simulink model "PRBS_Gen"  (R2019a)
settings: Solver=FixedStepAuto  StartTime=0.0  StopTime=TSim  FixedStep=0.2  RelTol=1e-3
values from neighbouring files (symbols this model uses):
  Num_Switch = 50    [MissionBlocks.m]    (also in Test.m = 1)
  Percent = 0.1    [MissionBlocks.m]    (also in Test.m)
  Samp_end = 2    [MissionBlocks.m]    (also in Test.m)
  Samp_start = 100    [MissionBlocks.m]    (also in Test.m)
  Samp_Switch = 2    [MissionBlocks.m]    (also in Test.m = 1000)
  Wf = [0.01335 0.01669 0.02 0.025 0.03 0.0334 0.04172 0.05 0.05841 0.06676]    [MissionBlocks.m]    (also in Test.m = WfMtx(2))
libraries: Lib_Solve_ModelSource_TMATS x1
settings Model: Creator=anton  LastModifiedBy=anton

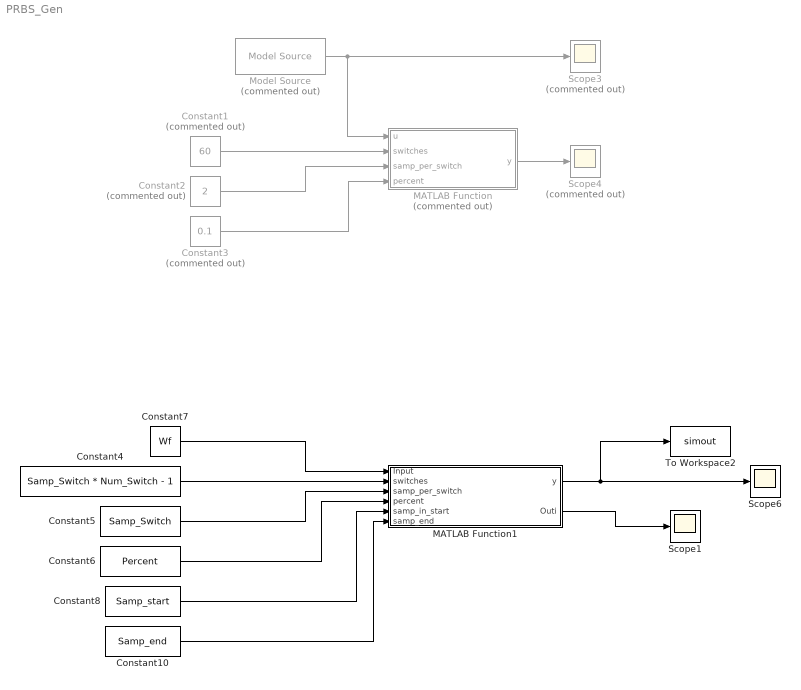
== system PRBS_Gen ==
  Constant1 : Constant  Commented=on  Value=60
  Constant10 : Constant  Value=Samp_end
  Constant2 : Constant  Commented=on  Value=2
  Constant3 : Constant  Commented=on  Value=0.1
  Constant4 : Constant  Value=Samp_Switch * Num_Switch - 1
  Constant5 : Constant  Value=Samp_Switch
  Constant6 : Constant  Value=Percent
  Constant7 : Constant  Value=Wf
  Constant8 : Constant  Value=Samp_start
  MATLAB Function : MATLAB Function  Commented=on  TreatAsAtomicUnit=on
  MATLAB Function1 : MATLAB Function  TreatAsAtomicUnit=on
  Model Source : Lib_Solve_ModelSource_TMATS/Model Source  Commented=on  T_vec_M=[0 15 15.1 30 30.1 45]  input_array_M=[5 5 10 10 15 15 ]
  Scope1 : Scope
  Scope3 : Scope  Commented=on
  Scope4 : Scope  Commented=on
  Scope6 : Scope
  To Workspace2 : ToWorkspace  VariableName=simout  SaveFormat=Timeseries  SampleTime=-1
  wires:
  Model Source/1 -> MATLAB Function/1(u), Scope3/1
  MATLAB Function/1(y) -> Scope4/1
  Constant1/1 -> MATLAB Function/2(switches)
  Constant2/1 -> MATLAB Function/3(samp_per_switch)
  Constant3/1 -> MATLAB Function/4(percent)
  Constant6/1 -> MATLAB Function1/4(percent)
  Constant5/1 -> MATLAB Function1/3(samp_per_switch)
  Constant4/1 -> MATLAB Function1/2(switches)
  MATLAB Function1/1(y) -> To Workspace2/1, Scope6/1
  Constant7/1 -> MATLAB Function1/1(Input)
  Constant8/1 -> MATLAB Function1/5(samp_in_start)
  Constant10/1 -> MATLAB Function1/6(samp_end)
  MATLAB Function1/2(Outi) -> Scope1/1

== matlab function PRBS_Gen/MATLAB Function1 ==
  settings: updateMethod=DISCRETE  sampleTime=0.2
  data: Input input; y output; switches input; samp_per_switch input; percent input; samp_in_start input; samp_end input; Outi output
function [y,Outi] = fcn(Input,switches,samp_per_switch,percent,samp_in_start,samp_end)
     
persistent state;
persistent u;
persistent switch_count;
persistent switch_stay;
persistent level_count;
persistent output

persistent i;

%Initiates outputs
y = Input(1);
LengIn = length(Input);
Outi = 0;

%Initiates persistent variables
if isempty(state)

    state = 0;
    switch_count = 0;
    switch_stay = 0;
    level_count = 1;
    output = Input(1);
    u = Input(1);
    i = 0;

    return;

end

switch state
    case 0
        %Updates output
        output = u;
        %Updates the number of samples of signal holding
        switch_stay = switch_stay + 1;
        %Verifies if signal has been held for enought sample periods
        if switch_stay == samp_in_start
            state = 1;
            switch_stay = samp_per_switch;
        end
    case 1
        %Verifies if signal has been held for enought sample periods
        if switch_stay == samp_per_switch && switch_count <= switches
            %Generates a random numver for coefficient generation
            coeff = rand(1,1);
            %Determines the coefficient for oscilation around input value
            if coeff > 0.5
                coeff = 1;
            else
                coeff = -1;
            end
            %Updates output
            output = u * (1 + coeff * percent);
            switch_stay = 0;
            i = i+1;
        end
        
        %Updates switch count
        switch_stay = switch_stay + 1;
        switch_count = switch_count + 1;
        
        %All switches have been accomplisehd
        if switch_count > switches
            state = 2;
            switch_stay = 0;
            switch_count = 0;
            i = 0;
        end
        
    case 2
        %If number of switches have been reached, the output must remain
        %equal current input level
        output = u;
        %Updates switch count
        switch_stay = switch_stay + 1;
        %If output is at current lavel for enough samples, next state is
        %activated
        if switch_stay >= samp_end
            state = 3;
            switch_stay = 0;
        end
        %If change is deteced, cycle starts again
    case 3
        %Updates signal level counter
        level_count = level_count + 1;
        %Updates u for next input level if possible
        if level_count <= LengIn
            u = Input(level_count);
            state = 0;
        end
        
end

%Updates fuel level for mission
y = output;
%Updates i - shows how many times the output is calculated while in prbs
Outi = i;

== matlab function PRBS_Gen/MATLAB Function ==
  settings: updateMethod=DISCRETE  sampleTime=0.2
  data: u input; y output; switches input; samp_per_switch input; percent input
function y = fcn(u,switches,samp_per_switch,percent)

persistent change;     %detects change in input
persistent state;
persistent switch_count;
persistent switch_stay;
persistent uk1
persistent output

y = 0;

if isempty(change)

    change = 1;
    state = 0;
    switch_count = 0;
    switch_stay = 0;
    uk1 = u;
    output = 0;

    return;

end



switch state
    case 0
        %Updates output
        output = u;
        %Updates the number of samples of signal holding
        switch_stay = switch_stay + 1;
        %Verifies if signal has been held for enought sample periods
        if switch_stay == samp_per_switch
            state = 1;
        end
    case 1
        %Verifies if signal has been held for enought sample periods
        if switch_stay == samp_per_switch && switch_count < switches
            %Generates a random numver for coefficient generation
            coeff = rand(1,1);
            %Determines the coefficient for oscilation around input value
            if coeff > 0.5
                coeff = 1;
            else
                coeff = -1;
            end
            %Updates output
            output = u * (1 + coeff * percent);
            switch_stay = 0;
        end
        
        if switch_count >= switches
            output = u;
        end
        %Updates switch count
        switch_stay = switch_stay + 1;
        switch_count = switch_count + 1;
        %If change is deteced, cycle starts again
        if u ~= uk1
            state = 0;
            switch_count = 0;
            switch_stay = 0;
        end
end

%Updates uk1 signal with current input values
uk1 = u;
%
y = output;
